simulink model "BloquesTransformacion"  (R2023a)
settings: Solver=VariableStepAuto  StartTime=0.0  StopTime=10.0  RelTol=1e-3
settings Model: Creator=juanf  LastModifiedBy=Juan

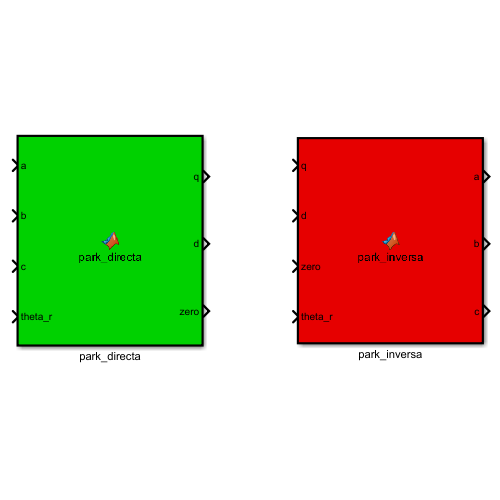
[thumbnail: Simulink's stored preview of the top-level diagram]
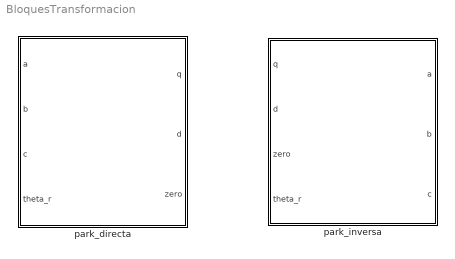
== system BloquesTransformacion ==
  park_directa : MATLAB Function  TreatAsAtomicUnit=on
  park_inversa : MATLAB Function  TreatAsAtomicUnit=on

== matlab function BloquesTransformacion/park_inversa ==
  data: q input; a output; d input; zero input; theta_r input; b output; c output
function [a, b, c] = park_inversa(q, d, zero, theta_r)
% qd0 → abc (transformacion inversa)
% Entradas: q, d, zero (coordenadas qd0), theta_r (ángulo eléctrico)
% Salidas: a, b, c (señales de fase)
    
    T_inv = [cos(theta_r),               sin(theta_r),              1;
             cos(theta_r - 2*pi/3),      sin(theta_r - 2*pi/3),     1;
             cos(theta_r + 2*pi/3),      sin(theta_r + 2*pi/3),     1];
    
    abc = T_inv * [q; d; zero];

    a = abc(1);
    b = abc(2);
    c = abc(3);
end

== matlab function BloquesTransformacion/park_directa ==
  data: a input; q output; b input; c input; theta_r input; d output; zero output
function [q, d, zero] = park_directa(a, b, c, theta_r)
% Transformacion abc → qd0
% a, b y c son señales de fase y theta_r es el angulo ELECTRICO (no mecanico) del rotor)
% Salidas: q, d, zero, que son las coordenadas virtuales qd0
    
    T = (2/3) * [cos(theta_r),           cos(theta_r - 2*pi/3),      cos(theta_r + 2*pi/3);
                 sin(theta_r),           sin(theta_r - 2*pi/3),      sin(theta_r + 2*pi/3);
                 1/2,                    1/2,                         1/2];
    
    qd0 = T * [a; b; c];
    
% asignar salidas
    q = qd0(1);
    d = qd0(2);
    zero = qd0(3);
end
